simulink model "phase_wrap_correction"  (R2013b)
settings: Solver=ode45  StartTime=0.0  StopTime=10.0  RelTol=1e-3
settings Model: Creator=aberger  LastModifiedBy=aberger

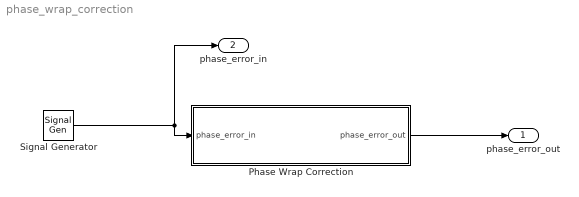
== system phase_wrap_correction ==
  Phase Wrap Correction : Subsystem
  Signal Generator : SignalGenerator  WaveForm=sawtooth
  phase_error_out : Outport
  phase_error_in : Outport  Port=2
  wires:
  Phase Wrap Correction/1(phase_error_out) -> phase_error_out/1
  Signal Generator/1 -> Phase Wrap Correction/1(phase_error_in), phase_error_in/1

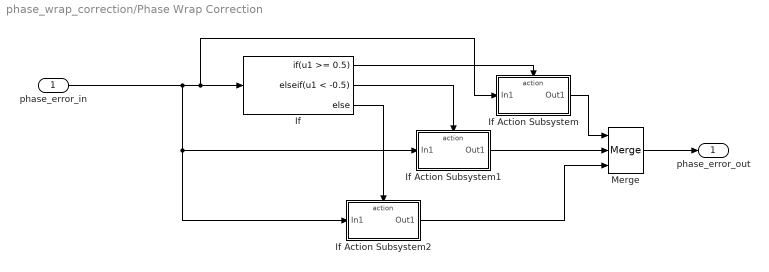
== system phase_wrap_correction/Phase Wrap Correction ==
  phase_error_in : Inport
  If : If  IfExpression=u1 >= 0.5  ElseIfExpressions=u1 < -0.5
  If Action Subsystem : Subsystem  TreatAsAtomicUnit=on
  If Action Subsystem1 : Subsystem  TreatAsAtomicUnit=on
  If Action Subsystem2 : Subsystem  TreatAsAtomicUnit=on
  Merge : Merge  Inputs=3
  phase_error_out : Outport
  wires:
  If/1 -> If Action Subsystem/Action
  If Action Subsystem/1(Out1) -> Merge/1
  If Action Subsystem2/1(Out1) -> Merge/3
  phase_error_in/1 -> If/1, If Action Subsystem/1(In1), If Action Subsystem1/1(In1), If Action Subsystem2/1(In1)
  If/2 -> If Action Subsystem1/Action
  If/3 -> If Action Subsystem2/Action
  Merge/1 -> phase_error_out/1
  If Action Subsystem1/1(Out1) -> Merge/2

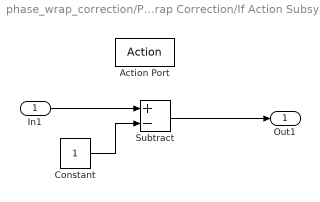
== system phase_wrap_correction/Phase Wrap Correction/If Action Subsystem ==
  In1 : Inport
  Action Port : ActionPort  ActionType=then
  Constant : Constant
  Subtract : Sum  Inputs=+-
  Out1 : Outport
  wires:
  In1/1 -> Subtract/1
  Constant/1 -> Subtract/2
  Subtract/1 -> Out1/1

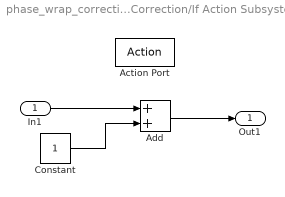
== system phase_wrap_correction/Phase Wrap Correction/If Action Subsystem1 ==
  In1 : Inport
  Action Port : ActionPort  ActionType=elseif
  Add : Sum
  Constant : Constant
  Out1 : Outport
  wires:
  In1/1 -> Add/1
  Constant/1 -> Add/2
  Add/1 -> Out1/1

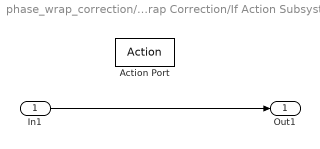
== system phase_wrap_correction/Phase Wrap Correction/If Action Subsystem2 ==
  In1 : Inport
  Action Port : ActionPort  ActionType=else
  Out1 : Outport
  wires:
  In1/1 -> Out1/1
